simulink model "Class_D_Amp"  (R2015b)
settings: Solver=FixedStepAuto  StartTime=0.0  StopTime=1e-3  RelTol=1e-3
values from neighbouring files (symbols this model uses):
  A = .5    (= 0.5)    [Class_D_Amp_Control.m]
  C = (1/(2*pi*f3dB)^2)*(1/L)    (= 5.23353221293e-08)    [Class_D_Amp_Control.m]
  DC = 0    [Class_D_Amp_Control.m]
  f_input = 10e3    (= 10000)    [Class_D_Amp_Control.m]
  Kamp = 5    [Class_D_Amp_Control.m]
  Ktri = 1    [Class_D_Amp_Control.m]
  L = 1e-3    (= 0.001)    [Class_D_Amp_Control.m]
  R = zeta/pi*sqrt(L/C)    [Class_D_Amp_Control.m]
libraries: simulink x1, powerlib_meascontrol x1
settings Model: Creator=Eric  LastModifiedBy=Eric

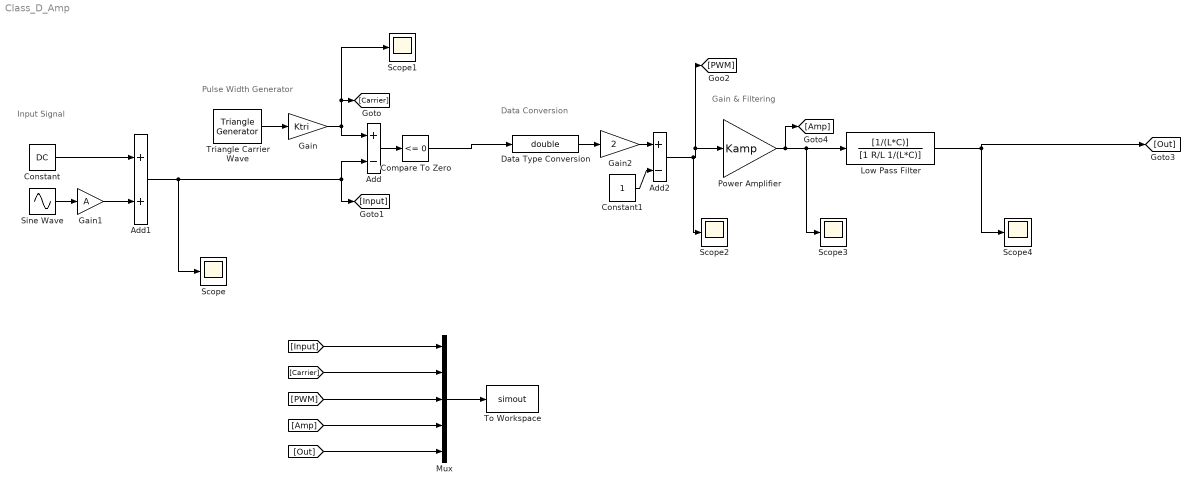
== system Class_D_Amp ==
  note: Data Conversion
  note: Input Signal
  note: Gain & Filtering
  note: Pulse Width Generator
  Add : Sum  Inputs=+-
  Add1 : Sum
  Add2 : Sum  Inputs=+-
  Compare To Zero : simulink/Logic and Bit Operations/Compare To Zero  relop=<=  OutDataTypeStr=boolean
  Constant : Constant  Value=DC
  Constant1 : Constant
  Data Type Conversion : DataTypeConversion  OutDataTypeStr=double
  Gain : Gain  Gain=Ktri
  Gain1 : Gain  Gain=A
  Gain2 : Gain  Gain=2
  Low Pass Filter : TransferFcn  Numerator=[1/(L*C)]  Denominator=[1 R/L 1/(L*C)]
  Mux : Mux  Inputs=5
  Power Amplifier : Gain  Gain=Kamp
  Scope{,1..4} (5 alike) : Scope
  Sine Wave : Sin  Frequency=2*pi*f_input  SampleTime=0
  To Workspace : ToWorkspace  VariableName=simout  SaveFormat=Structure With Time  SampleTime=-1
  Triangle Carrier Wave : powerlib_meascontrol/Pulse & Signal Generators/Triangle Generator  Freq=f_tri  Phase=90  Ts=0
  wires:
  Add/1 -> Compare To Zero/1
  Triangle Carrier Wave/1 -> Gain/1
  Gain/1 -> Scope1/1, [Carrier], Add/1
  Compare To Zero/1 -> Data Type Conversion/1
  Power Amplifier/1 -> [Amp], Scope3/1, Low Pass Filter/1
  Sine Wave/1 -> Gain1/1
  Constant/1 -> Add1/1
  Gain1/1 -> Add1/2
  Low Pass Filter/1 -> [Out], Scope4/1
  [Input] -> Mux/1
  [Carrier] -> Mux/2
  [Amp] -> Mux/4
  [Out] -> Mux/5
  Mux/1 -> To Workspace/1
  [PWM] -> Mux/3
  Add1/1 -> Scope/1, [Input], Add/2
  Data Type Conversion/1 -> Gain2/1
  Constant1/1 -> Add2/2
  Gain2/1 -> Add2/1
  Add2/1 -> Scope2/1, [PWM], Power Amplifier/1
